simulink model "RobotX_SLAMonly"  (R2014a)
settings: Solver=FixedStepDiscrete  StartTime=0.0  StopTime=inf  FixedStep=.25  RelTol=1e-3
undefined symbols (not defined in the file): Com1, Com2, Com3, Com4, DiscIntNeverNeededParam, standard
libraries: xpcseriallib x11, simulink x3, slrtlib x3, dspmtrx3 x2, speedgoatlib x1, speedgoatlib_IO102 x1
(part 1 of 15)
settings Model: BufferReuse=off  Creator=wildcat  LastModifiedBy=wildcat
settings SolverCC: EnableConcurrentExecution=on
settings DataIOCC: SignalLoggingSaveFormat=ModelDataLogs
settings OptimizationCC: BlockReduction=off  OptimizeBlockIOStorage=off  BufferReuse=off  GlobalBufferReuse=off  ExpressionFolding=off  LocalBlockOutputs=off
settings DebuggingCC: UnderspecifiedInitializationDetection=Classic  StateNameClashWarn=warning
settings HardwareCC: ProdIntDivRoundTo=Zero  ProdEndianess=LittleEndian  ProdHWDeviceType=Generic->32-bit x86 compatible
settings RTWCC: SystemTargetFile=slrt.tlc  TemplateMakefile=slrt_default_tmf  Description=Simulink Real-Time  ProcessScript=slrt_make_rtw_hook  RTWCompilerOptimization=On
settings SimulinkRealTimeCC: GeneratePreprocessorConditionals=Disable all  EnableShiftOperators=on

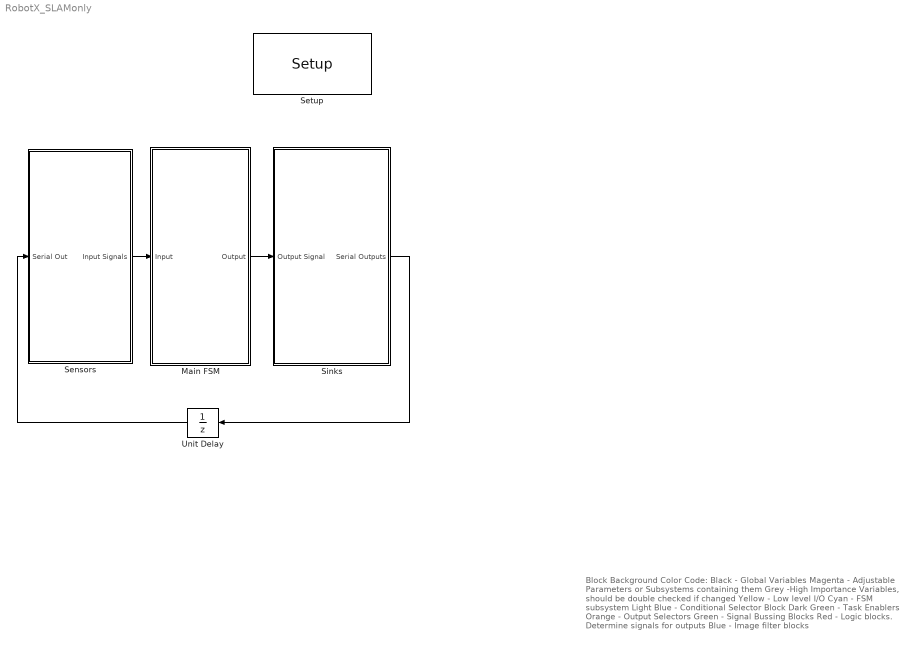
== system RobotX_SLAMonly ==
  note: Block Background Color Code:
      | Black - Global Variables
      | Magenta - Adjustable Parameters or Subsystems containing them
      | Grey -High Importance Variables, should be double checked if changed
      | Yellow - Low level I/O
      | Cyan - FSM subsystem
      | Light Blue - Conditional Selector Block
      | Dark Green - Task Enablers
      | Orange - Output Selectors
      | Green - Signal Bussing Blocks
      | Red - Logic blocks. Determine signals for outputs
      | Blue - Image filter blocks
  Main FSM : Subsystem
  Sensors : Subsystem
  Setup : speedgoatlib_IO102/Setup  group=Digital output setup  id=1  range=+-5V  cal=off  pciSlot=-1  adChannelMode=Multiple-channel (enter number of channels below)  adChannel=16  adCoupling=Differential  daChannel=[1,2,3,4]  daReset=[1]  daInitValue=[0]  diChannel=[1,2,3,4,5,6,7,8]  doChannel=[1,2,3,4,5,6,7,8]  doReset=[1]  doInitValue=[0]
  Sinks : Subsystem
  Unit Delay : UnitDelay  SampleTime=-1
  wires:
  Main FSM/1(Output) -> Sinks/1(Output Signal)
  Sensors/1(Input Signals) -> Main FSM/1(Input)
  Sinks/1(Serial Outputs) -> Unit Delay/1
  Unit Delay/1 -> Sensors/1(Serial Out)

== system RobotX_SLAMonly/Main FSM ==
  Input : Inport
  Angles : dspmtrx3/Submatrix  RowSpan=All rows  RowStartMode=First  RowStartIndex=1  RowEndMode=Last  RowEndIndex=1  ColSpan=One column  ColStartMode=Last  ColStartIndex=1  ColEndMode=Last  ColEndIndex=1
  Bus Selector2 : BusSelector  OutputSignals=Navigation Message.On/Off/RC/Auto
  Distances : dspmtrx3/Submatrix  RowSpan=All rows  RowStartMode=First  RowStartIndex=1  RowEndMode=Last  RowEndIndex=1  ColSpan=One column  ColStartMode=First  ColStartIndex=1  ColEndMode=Last  ColEndIndex=1
  Initialization : Subsystem
  Main Enabler : MATLAB Function  TreatAsAtomicUnit=on
  Multiport Switch : MultiPortSwitch
  Path : Subsystem  TreatAsAtomicUnit=on
  RCHold : Subsystem
  SLAM : Subsystem
  "Scope " : slrtlib/Displays and Logging/Scope   scopeno=1  scopetype=File  autostart=on  viewmode=Graphical redraw  formatstr='%15.6f'  grid=on  ylimits=[0,0]  nosamples=28800  noprepostsamples=0  interleave=1  triggermode=FreeRun  triggersignal=1  trigsignalfromport=off  triggerlevel=0.0  triggerslope=Either  triggerscope=1  triggersample=0  filename=lmD1_<%%%>.dat  mode=Lazy  writesize=512  autorestart=on  dynamicfilemode=on  maxwritefilesize=512*1024^2
  Scope 1 : slrtlib/Displays and Logging/Scope   scopeno=2  scopetype=File  autostart=on  viewmode=Graphical redraw  formatstr='%15.6f'  grid=on  ylimits=[0,0]  nosamples=28800  noprepostsamples=0  interleave=1  triggermode=FreeRun  triggersignal=1  trigsignalfromport=off  triggerlevel=0.0  triggerslope=Either  triggerscope=1  triggersample=0  filename=lmA1_<%%%>.dat  mode=Lazy  writesize=512  autorestart=on  dynamicfilemode=on  maxwritefilesize=512*1024^2
  Unit Delay : UnitDelay  SampleTime=-1
  Output : Outport
  wires:
  Input/1 -> SLAM/1(Sensors), Path/1(Sensors), RCHold/1(Sensors), Initialization/1(Sensors), Bus Selector2/1
  Bus Selector2/1 -> Main Enabler/1(OnOffRCAuto)  "<On/Off/RC/Auto>"
  Initialization/1(Outputs) -> Multiport Switch/2
  Path/1(Outputs) -> Multiport Switch/3
  RCHold/1(Outputs) -> Multiport Switch/4
  Main Enabler/2(initEn) -> Initialization/Enable
  Main Enabler/3(pathEn) -> Path/Enable
  Main Enabler/4(RCEn) -> RCHold/Enable
  Main Enabler/1(taskSelector) -> Multiport Switch/1
  Multiport Switch/1 -> Output/1
  Initialization/2(Finished) -> Unit Delay/1  "Init Fin"
  Unit Delay/1 -> Main Enabler/2(initFin)
  SLAM/1(SLAM Map) -> Angles/1, Distances/1
  Distances/1 -> "Scope "/1
  Angles/1 -> Scope 1/1

== system RobotX_SLAMonly/Sensors ==
  Serial Out : Inport
  Serial In : Subsystem
  Input Signals : Outport
  wires:
  Serial In/1(Serial In) -> Input Signals/1  "Sensors"
  Serial Out/1 -> Serial In/1(Serial Out)

== system RobotX_SLAMonly/Sinks ==
  Output Signal : Inport
  Bus Selector : BusSelector  OutputSignals=Outputs
  data log : Subsystem  Commented=on
  Serial Outputs : Outport
  wires:
  Output Signal/1 -> Bus Selector/1
  Bus Selector/1 -> Serial Outputs/1  "<Outputs>"

== system RobotX_SLAMonly/Main FSM/Initialization ==
  Sensors : Inport
  Enable : EnablePort  ShowOutputPort=on
  Compare To Constant : simulink/Logic and Bit Operations/Compare To Constant  relop=>=  const=50  OutDataTypeStr=boolean
  Data Type Conversion : DataTypeConversion  OutDataTypeStr=double
  Discrete-Time Integrator : DiscreteIntegrator  SampleTime=-1  ICPrevOutput=DiscIntNeverNeededParam  ICPrevScaledInput=DiscIntNeverNeededParam
  Output Heirarchy : Subsystem
  Outputs : Outport
  Finished : Outport  Port=2
  wires:
  Sensors/1 -> Output Heirarchy/1(Sensors)
  Output Heirarchy/1(Outputs) -> Outputs/1
  Compare To Constant/1 -> Data Type Conversion/1
  Enable/1 -> Discrete-Time Integrator/1
  Discrete-Time Integrator/1 -> Compare To Constant/1
  Data Type Conversion/1 -> Finished/1

== system RobotX_SLAMonly/Main FSM/Path ==
  note: Through Gate
  Sensors : Inport
  Enable : EnablePort  ShowOutputPort=on
  A Star (Held Length) : MATLAB Function  TreatAsAtomicUnit=on
  Bus Selector : BusSelector  OutputSignals=Navigation Message.Pose.X,Navigation Message.Pose.Y,Navigation Message.Pose.Psi
  Bus Selector1 : BusSelector  OutputSignals=Navigation Message.Velocity.u
  Calculate Times : MATLAB Function  TreatAsAtomicUnit=on
  Constant : Constant  Value=3
  Constant1 : Constant  Value=[3558, 662; 3625, 652; 3577, 568; 3614, 558]
  Constant2 : Constant  Value=[10, 5; 15, 26; 28, 19; 15, 8; 50, 30]
  Discrete-Time Integrator : DiscreteIntegrator  SampleTime=-1  ICPrevOutput=DiscIntNeverNeededParam  ICPrevScaledInput=DiscIntNeverNeededParam
  Map Grid (Held Length) : MATLAB Function  TreatAsAtomicUnit=on
  Output Reassign : Subsystem
  Path To Trajectory : MATLAB Function  TreatAsAtomicUnit=on
  Outputs : Outport
  wires:
  Output Reassign/1(Outputs) -> Outputs/1
  Enable/1 -> Discrete-Time Integrator/1
  Map Grid (Held Length)/1(relPose) -> A Star (Held Length)/1(relPose), Path To Trajectory/2(relPose)
  Map Grid (Held Length)/2(obGrid) -> A Star (Held Length)/2(obGrid)
  Map Grid (Held Length)/3(targetPt) -> A Star (Held Length)/3(targetPt)
  A Star (Held Length)/1(Path) -> Path To Trajectory/3(Path)
  Map Grid (Held Length)/4(nodes) -> Path To Trajectory/4(nodes)
  Constant/1 -> Map Grid (Held Length)/1(exitGate)
  Constant1/1 -> Map Grid (Held Length)/2(NEDcorners)
  Bus Selector/2 -> Map Grid (Held Length)/4(Y)  "<Y>"
  Bus Selector/3 -> Map Grid (Held Length)/5(Psi)  "<Psi>"
  Constant2/1 -> Map Grid (Held Length)/6(NEDlandmarks)
  Bus Selector/1 -> Map Grid (Held Length)/3(X)  "<X>"
  Path To Trajectory/2(trajectory) -> Calculate Times/1(pts)
  Bus Selector1/1 -> Calculate Times/2(u)  "<u>"
  Path To Trajectory/1(valid) -> Output Reassign/1("Valid ")
  Calculate Times/1(Data) -> Output Reassign/2(Data)
  Sensors/1 -> Output Reassign/3(Sensors), Bus Selector1/1, Bus Selector/1
  Discrete-Time Integrator/1 -> Path To Trajectory/1(time)

== system RobotX_SLAMonly/Main FSM/RCHold ==
  Sensors : Inport
  Enable : EnablePort
  Bus Selector : BusSelector  Commented=on  OutputSignals=LCM Message.Pose.X,LCM Message.Pose.Y,LCM Message.Pose.Psi
  Output Heirarchy : Subsystem  Commented=on
  Output Heirarchy1 : Subsystem
  Set Pose : MATLAB Function  Commented=on  TreatAsAtomicUnit=on
  Outputs : Outport
  wires:
  Output Heirarchy1/1(Outputs) -> Outputs/1
  Bus Selector/1 -> Set Pose/1(X)  "<X>"
  Bus Selector/3 -> Set Pose/3(Psi)  "<Psi>"
  Bus Selector/2 -> Set Pose/2(Y)  "<Y>"
  Set Pose/1(Data) -> Output Heirarchy/1(Data)
  Sensors/1 -> Output Heirarchy1/1(Sensors), Bus Selector/1

== system RobotX_SLAMonly/Main FSM/SLAM ==
  Sensors : Inport
  Any Landmark Change : MATLAB Function  TreatAsAtomicUnit=on
  Any State Change : MATLAB Function  TreatAsAtomicUnit=on
  Bus Selector : BusSelector  OutputSignals=Navigation Message,Lidar Data Input
  Bus Selector1 : BusSelector  OutputSignals=Landmarks.Distances,Landmarks.Angles
  Bus Selector2 : BusSelector  OutputSignals=Pose
  Detect Change : simulink/Logic and Bit Operations/Detect Change  vinit=0  InputProcessing=Inherited  OutDataTypeStr=boolean
  Detect Change1 : simulink/Logic and Bit Operations/Detect Change  vinit=0  InputProcessing=Inherited  OutDataTypeStr=boolean
  Landmark Organizer : MATLAB Function  TreatAsAtomicUnit=on
  Models for prediction : Subsystem
  SLAM enabled : Subsystem  TreatAsAtomicUnit=on
  inputselection : Subsystem
  SLAM Map : Outport
  wires:
  Sensors/1 -> Bus Selector/1
  Bus Selector/1 -> Models for prediction/1(Nav Messages), Bus Selector2/1, Detect Change/1  "<Navigation Message>"
  Bus Selector/2 -> Bus Selector1/1  "<Lidar Data Input>"
  Bus Selector1/1 -> Landmark Organizer/1(Distances)  "<Distances>"
  Bus Selector1/2 -> Landmark Organizer/2(Angles)  "<Angles>"
  Landmark Organizer/1(lm_data) -> SLAM enabled/2(lm_data), Detect Change1/1
  Detect Change/1 -> Any State Change/1(u)
  Detect Change1/1 -> Any Landmark Change/1(u)
  Any Landmark Change/1(y) -> SLAM enabled/Enable, inputselection/3(Landmarkchange)
  Bus Selector2/1 -> inputselection/2(xypsi)  "<Pose>"
  Any State Change/1(y) -> inputselection/1(controlchange)
  SLAM enabled/2(part_positions) -> inputselection/4(part_positions)
  inputselection/1(last particle positions) -> Models for prediction/2(xypsi150)
  Models for prediction/1(xypsioutput) -> inputselection/5(xypsi150), SLAM enabled/1(pre_past_positions)
  SLAM enabled/1(mpa) -> SLAM Map/1  "SLAM Map"

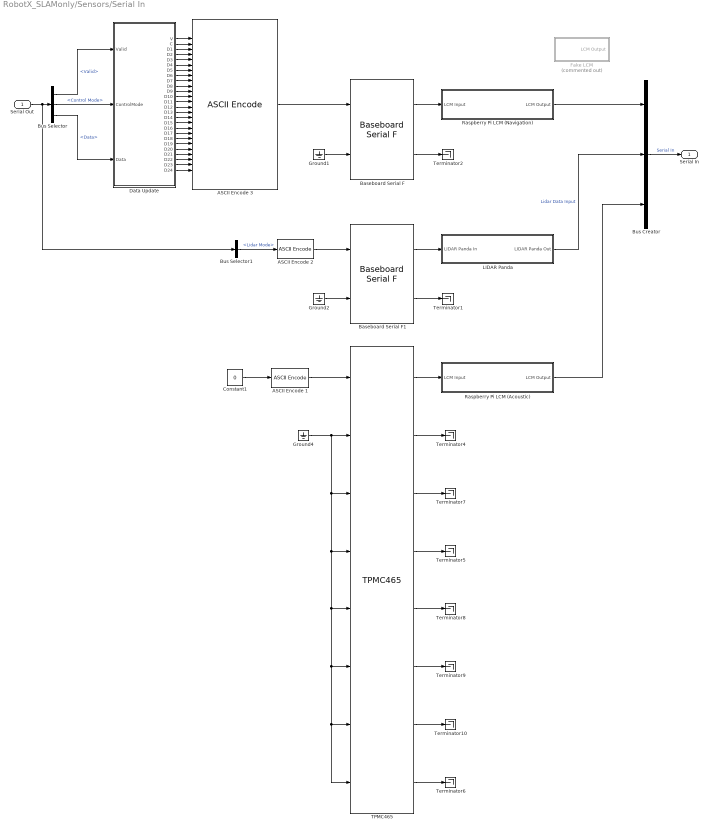
== system RobotX_SLAMonly/Sensors/Serial In ==
  Serial Out : Inport
  " Raspberry Pi LCM (Acoustic)" : Subsystem
  " Raspberry Pi LCM (Navigation)" : Subsystem
  ASCII Encode 1 : xpcseriallib/ASCII Encode   format="{\"Activate\":%d} \\r\\n"  nvars=1  maxlength=20  vartypes={ 'double' }
  ASCII Encode 2 : xpcseriallib/ASCII Encode   format=SGTask:%d \r\n  nvars=1  maxlength=128  vartypes={ 'double' }
  ASCII Encode 3 : xpcseriallib/ASCII Encode   format="{\"Valid\":%d,\"Mode\":%d,\"A\":%f,\"B\":%f,\"C\":%f,\"D\":%f,\"E\":%f,\"F\":%f,\"G\":%f,\"H\":%f,\"I\":%f,\"J\":%f,\"K\":%f,\"L\":%f,\"M\":%f,\"N\":%f,\"O\":%f,\"P\":%f,\"Q\":%f,\"R\":%f,\"S\":%f,\"T\":%f,\"U\":%f,\"V\":%f,\"W\":%f,\"X\":%f} \\r\\n"  nvars=26  maxlength=450  vartypes={ 'double' }
  Baseboard Serial F : xpcseriallib/Mainboard/Baseboard Serial F  group=Basic Setup  port=1  irqnum=4  saddr1=0x3f8  saddr2=0x3e8  config=Com1/Com3  baud1=115200  parity1=Even  ndata1=7  nstop1=1  fifomode1=64 deep  rlevel1=quarter full  automode1=on  xmtfifosize1=1024  xmtdatatype1=8 bit uint null terminated  rcvfifosize1=1024  baud2=115200  parity2=Even  ndata2=7  nstop2=1  fifomode2=64 deep  rlevel2=1  automode2=on  xmtfifosize2=1024  xmtdatatype2=8 bit uint null terminated  rcvfifosize2=1024
  Baseboard Serial F1 : xpcseriallib/Mainboard/Baseboard Serial F  group=Basic Setup  port=2  irqnum=4  saddr1=0x3f8  saddr2=0x3e8  config=Com2/Com4  baud1=115200  parity1=Even  ndata1=7  nstop1=1  fifomode1=64 deep  rlevel1=quarter full  automode1=on  xmtfifosize1=1024  xmtdatatype1=8 bit uint null terminated  rcvfifosize1=1024  baud2=115200  parity2=Even  ndata2=7  nstop2=1  fifomode2=64 deep  rlevel2=quarter full  automode2=on  xmtfifosize2=1024  xmtdatatype2=8 bit uint null terminated  rcvfifosize2=1024
  Bus Creator : BusCreator  Inputs=3
  Bus Selector : BusSelector  OutputSignals=Navigation Outputs.Valid,Navigation Outputs.Control Mode,Navigation Outputs.Data
  Bus Selector1 : BusSelector  OutputSignals=Lidar Mode
  Constant1 : Constant  Value=0  VectorParams1D=off
  Data Update : MATLAB Function  TreatAsAtomicUnit=on
  Fake LCM : Subsystem  Commented=on
  Ground1 : Ground
  Ground2 : Ground
  Ground4 : Ground
  LIDAR Panda : Subsystem
  TPMC465 : speedgoatlib/IO504/TPMC465  group=Basic Setup  port=2  irqnum=9  slot=-1  transceiver1=RS232 (max 921.6kb/s)  standard1=on  baud1=115200  bauddivisor1=1  sampling1=16x (standard)  prescale1=off  parity1=Even  ndata1=7  nstop1=1  rlevel1=half full (32)  hwmode1=none  swmode1=none  xonchar1=17  xoffchar1=19  rs485auto1=off  rs485delay1=0  xmtfifosize1=1024  xmtdatatype1=8 bit uint null terminated  rcvfifosize1=1024  transceiver2=RS232 (max 921.6kb/s)  standard2=on  baud2=115200  bauddivisor2=1  sampling2=16x (standard)  prescale2=off  parity2=None  ndata2=8  nstop2=1  rlevel2=half full (32)  hwmode2=none  swmode2=none  xonchar2=17  xoffchar2=19  rs485auto2=off  rs485delay2=0  xmtfifosize2=1024  xmtdatatype2=8 bit uint null terminated  rcvfifosize2=1024  transceiver3=RS232 (max 921.6kb/s)  standard3=on  baud3=115200  bauddivisor3=1  sampling3=16x (standard)  prescale3=off  parity3=None  ndata3=8  nstop3=1  rlevel3=half full (32)  hwmode3=none  swmode3=none  xonchar3=17  xoffchar3=19  rs485auto3=off  rs485delay3=0  xmtfifosize3=1024  xmtdatatype3=8 bit uint null terminated  rcvfifosize3=1024  transceiver4=RS232 (max 921.6kb/s)  standard4=on  baud4=115200  bauddivisor4=1  sampling4=16x (standard)  prescale4=off  parity4=None  ndata4=8  nstop4=1  rlevel4=half full (32)  hwmode4=none  swmode4=none  xonchar4=17  xoffchar4=19  rs485auto4=off  rs485delay4=0  xmtfifosize4=1024  xmtdatatype4=8 bit uint null terminated  rcvfifosize4=1024  transceiver5=RS232 (max 921.6kb/s)  standard5=on  baud5=115200  bauddivisor5=1  sampling5=16x (standard)  prescale5=off  parity5=None  ndata5=8  nstop5=1  rlevel5=1  hwmode5=none  swmode5=none  xonchar5=17  xoffchar5=19  rs485auto5=off  rs485delay5=0  xmtfifosize5=1024  xmtdatatype5=8 bit uint null terminated  rcvfifosize5=1024  transceiver6=RS232 (max 921.6kb/s)  standard6=on  baud6=115200  bauddivisor6=1  sampling6=16x (standard)  prescale6=off  parity6=None  ndata6=8  nstop6=1  rlevel6=1  hwmode6=none  swmode6=none  xonchar6=17  xoffchar6=19  rs485auto6=off  rs485delay6=0  xmtfifosize6=1024  xmtdatatype6=8 bit uint null terminated  rcvfifosize6=1024  transceiver7=RS232 (max 921.6kb/s)  standard7=on  baud7=115200  bauddivisor7=1  sampling7=16x (standard)  prescale7=off  parity7=None  ndata7=8  nstop7=1  rlevel7=1  hwmode7=none  swmode7=none  xonchar7=17  xoffchar7=19  rs485auto7=off  rs485delay7=0  xmtfifosize7=1024  xmtdatatype7=8 bit uint null terminated  rcvfifosize7=1024  transceiver8=RS232 (max 921.6kb/s)  standard8=on  baud8=115200  bauddivisor8=1  sampling8=16x (standard)  prescale8=off  parity8=None  ndata8=8  nstop8=1  rlevel8=1  hwmode8=none  swmode8=none  xonchar8=17  xoffchar8=19  rs485auto8=off  rs485delay8=0  xmtfifosize8=1024  xmtdatatype8=8 bit uint null terminated  rcvfifosize8=1024
  Terminator{1..2,4..10} (9 alike) : Terminator
  Serial In : Outport
  wires:
  Bus Creator/1 -> Serial In/1  "Serial In"
  Baseboard Serial F1/1 -> LIDAR Panda/1(LIDAR Panda In)
  Serial Out/1 -> Bus Selector1/1, Bus Selector/1
  Baseboard Serial F/1 -> " Raspberry Pi LCM (Navigation)"/1(LCM Input)
  TPMC465/1 -> " Raspberry Pi LCM (Acoustic)"/1(LCM Input)
  ASCII Encode 3/1 -> Baseboard Serial F/1
  " Raspberry Pi LCM (Navigation)"/1(LCM Output) -> Bus Creator/1
  ASCII Encode 1/1 -> TPMC465/1
  Data Update/9(D7) -> ASCII Encode 3/9
  Data Update/11(D9) -> ASCII Encode 3/11
  Data Update/3(D1) -> ASCII Encode 3/3
  Data Update/6(D4) -> ASCII Encode 3/6
  Data Update/7(D5) -> ASCII Encode 3/7
  Data Update/2(C) -> ASCII Encode 3/2
  Data Update/5(D3) -> ASCII Encode 3/5
  Data Update/4(D2) -> ASCII Encode 3/4
  Data Update/13(D11) -> ASCII Encode 3/13
  Data Update/14(D12) -> ASCII Encode 3/14
  Data Update/1(V) -> ASCII Encode 3/1
  Data Update/12(D10) -> ASCII Encode 3/12
  Data Update/10(D8) -> ASCII Encode 3/10
  Data Update/8(D6) -> ASCII Encode 3/8
  Bus Selector/1 -> Data Update/1(Valid)  "<Valid>"
  Bus Selector/2 -> Data Update/2(ControlMode)  "<Control Mode>"
  Bus Selector/3 -> Data Update/3(Data)  "<Data>"
  Data Update/24(D22) -> ASCII Encode 3/24
  Data Update/26(D24) -> ASCII Encode 3/26
  Data Update/18(D16) -> ASCII Encode 3/18
  Data Update/23(D21) -> ASCII Encode 3/23
  Data Update/22(D20) -> ASCII Encode 3/22
  Data Update/21(D19) -> ASCII Encode 3/21
  Data Update/19(D17) -> ASCII Encode 3/19
  Data Update/17(D15) -> ASCII Encode 3/17
  Data Update/16(D14) -> ASCII Encode 3/16
  Data Update/25(D23) -> ASCII Encode 3/25
  Data Update/20(D18) -> ASCII Encode 3/20
  Data Update/15(D13) -> ASCII Encode 3/15
  " Raspberry Pi LCM (Acoustic)"/1(LCM Output) -> Bus Creator/3
  Baseboard Serial F/2 -> Terminator2/1
  Ground1/1 -> Baseboard Serial F/2
  ASCII Encode 2/1 -> Baseboard Serial F1/1
  LIDAR Panda/1(LIDAR Panda Out) -> Bus Creator/2  "Lidar Data Input"
  TPMC465/7 -> Terminator10/1
  TPMC465/5 -> Terminator8/1
  TPMC465/6 -> Terminator9/1
  TPMC465/3 -> Terminator7/1
  TPMC465/2 -> Terminator4/1
  TPMC465/4 -> Terminator5/1
  TPMC465/8 -> Terminator6/1
  Ground4/1 -> TPMC465/2, TPMC465/3, TPMC465/4, TPMC465/5, TPMC465/6, TPMC465/7, TPMC465/8
  Baseboard Serial F1/2 -> Terminator1/1
  Ground2/1 -> Baseboard Serial F1/2
  Bus Selector1/1 -> ASCII Encode 2/1  "<Lidar Mode>"
  Constant1/1 -> ASCII Encode 1/1

== system RobotX_SLAMonly/Sinks/data log ==
  note: need to play with the boat to figure out how this works properly
  Output signal : Inport
  "Scope " : slrtlib/Displays and Logging/Scope   scopeno=1  scopetype=File  autostart=on  viewmode=Graphical redraw  formatstr='%15.6f'  grid=on  ylimits=[0,0]  nosamples=250  noprepostsamples=0  interleave=1  triggermode=Signal triggering  triggersignal=1  trigsignalfromport=on  triggerlevel=1  triggerslope=Rising  triggerscope=1  triggersample=0  filename=data.dat  mode=Lazy  writesize=512  autorestart=off  dynamicfilemode=off  maxwritefilesize=512*1024^2
  wires:
  Output signal/1 -> ?

== system RobotX_SLAMonly/Main FSM/Initialization/Output Heirarchy ==
  Sensors : Inport
  Acoustic Active : Constant  Value=0
  Bus Creator1 : BusCreator  Inputs=3
  Bus Creator2 : BusCreator  Inputs=3
  Bus Creator4 : BusCreator  Inputs=2
  Constant : Constant  Value=0
  Constant1 : Constant  Value=0
  Constant2 : Constant  Value=zeros(24,1)
  Lidar Mode : Constant  Value=0
  Outputs : Outport
  wires:
  Sensors/1 -> Bus Creator4/2  "Sensors"
  Bus Creator4/1 -> Outputs/1  "Output Signals"
  Constant/1 -> Bus Creator1/1  "Valid"
  Constant1/1 -> Bus Creator1/2  "Control Mode"
  Constant2/1 -> Bus Creator1/3  "Data"
  Bus Creator1/1 -> Bus Creator2/1  "Navigation Outputs"
  Acoustic Active/1 -> Bus Creator2/2  "Acoustic Active"
  Lidar Mode/1 -> Bus Creator2/3  "Lidar Mode"
  Bus Creator2/1 -> Bus Creator4/1  "Outputs"

== system RobotX_SLAMonly/Main FSM/Path/Output Reassign ==
  "Valid " : Inport
  Data : Inport  Port=2
  Sensors : Inport  Port=3
  Acoustic Active : Constant
  Bus Creator2 : BusCreator  Inputs=3
  Bus Creator3 : BusCreator  Inputs=3
  Bus Creator5 : BusCreator  Inputs=2
  Constant3 : Constant
  Lidar Mode : Constant
  Outputs : Outport
  wires:
  Sensors/1 -> Bus Creator5/2  "Sensors"
  Bus Creator5/1 -> Outputs/1  "Output Signals"
  "Valid "/1 -> Bus Creator2/1  "Valid"
  Constant3/1 -> Bus Creator2/2  "Control Mode"
  Data/1 -> Bus Creator2/3  "Data"
  Bus Creator2/1 -> Bus Creator3/1  "Navigation Outputs"
  Acoustic Active/1 -> Bus Creator3/2  "Acoustic Active"
  Lidar Mode/1 -> Bus Creator3/3  "Lidar Mode"
  Bus Creator3/1 -> Bus Creator5/1  "Outputs"

== system RobotX_SLAMonly/Main FSM/RCHold/Output Heirarchy ==
  Data : Inport
  Sensors1 : Inport  Port=2
  Acoustic Active : Constant  Value=0
  Bus Creator2 : BusCreator  Inputs=3
  Bus Creator3 : BusCreator  Inputs=3
  Bus Creator5 : BusCreator  Inputs=2
  Constant : Constant
  Constant3 : Constant
  Lidar Mode : Constant
  Outputs : Outport
  wires:
  Sensors1/1 -> Bus Creator5/2  "Sensors"
  Bus Creator5/1 -> Outputs/1  "Output Signals"
  Constant/1 -> Bus Creator2/1  "Valid"
  Constant3/1 -> Bus Creator2/2  "Control Mode"
  Data/1 -> Bus Creator2/3  "Data"
  Bus Creator2/1 -> Bus Creator3/1  "Navigation Outputs"
  Acoustic Active/1 -> Bus Creator3/2  "Acoustic Active"
  Lidar Mode/1 -> Bus Creator3/3  "Lidar Mode"
  Bus Creator3/1 -> Bus Creator5/1  "Outputs"

== system RobotX_SLAMonly/Main FSM/RCHold/Output Heirarchy1 ==
  Sensors : Inport
  Acoustic Active : Constant  Value=0
  Bus Creator1 : BusCreator  Inputs=3
  Bus Creator2 : BusCreator  Inputs=3
  Bus Creator4 : BusCreator  Inputs=2
  Constant : Constant  Value=0
  Constant1 : Constant  Value=2
  Constant2 : Constant  Value=zeros(24,1)
  Lidar Mode : Constant
  Outputs : Outport
  wires:
  Sensors/1 -> Bus Creator4/2  "Sensors"
  Bus Creator4/1 -> Outputs/1  "Output Signals"
  Constant/1 -> Bus Creator1/1  "Valid"
  Constant1/1 -> Bus Creator1/2  "Control Mode"
  Constant2/1 -> Bus Creator1/3  "Data"
  Bus Creator1/1 -> Bus Creator2/1  "Navigation Outputs"
  Acoustic Active/1 -> Bus Creator2/2  "Acoustic Active"
  Lidar Mode/1 -> Bus Creator2/3  "Lidar Mode"
  Bus Creator2/1 -> Bus Creator4/1  "Outputs"

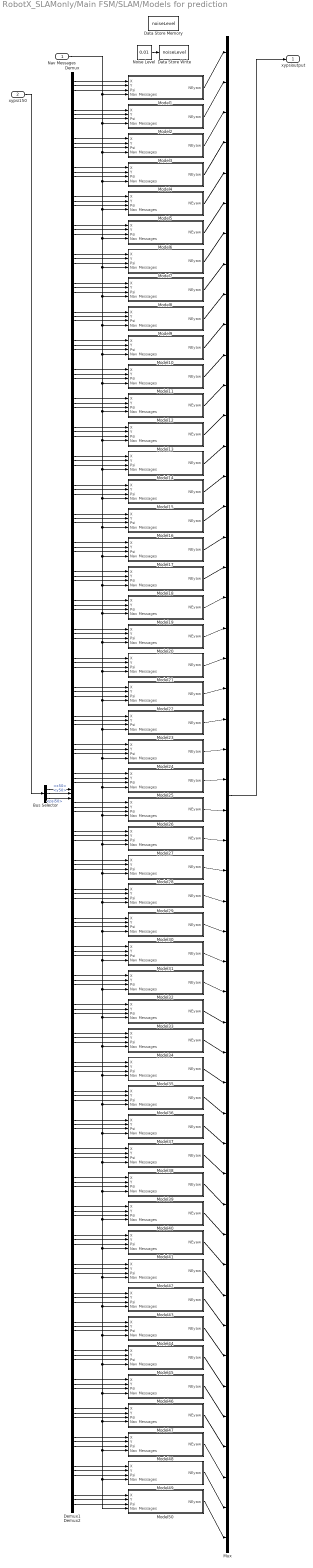
== system RobotX_SLAMonly/Main FSM/SLAM/Models for prediction ==
  Nav Messages : Inport
  xypsi150 : Inport  Port=2
  Bus Selector : BusSelector  OutputSignals=x50,y50,psi50
  Data Store Memory : DataStoreMemory  DataStoreName=noiseLevel  ReadBeforeWriteMsg=warning  WriteAfterWriteMsg=warning  WriteAfterReadMsg=warning
  Data Store Write : DataStoreWrite  DataStoreName=noiseLevel
  Demux : Demux  Outputs=50
  Demux1 : Demux  Outputs=50
  Demux2 : Demux  Outputs=50
  Model1 : Subsystem
  Model10 : Subsystem
  Model11 : Subsystem
  Model12 : Subsystem
  Model13 : Subsystem
  Model14 : Subsystem
  Model15 : Subsystem
  Model16 : Subsystem
  Model17 : Subsystem
  Model18 : Subsystem
  Model19 : Subsystem
  Model2 : Subsystem
  Model20 : Subsystem
  Model21 : Subsystem
  Model22 : Subsystem
  Model23 : Subsystem
  Model24 : Subsystem
  Model25 : Subsystem
  Model26 : Subsystem
  Model27 : Subsystem
  Model28 : Subsystem
  Model29 : Subsystem
  Model3 : Subsystem
  Model30 : Subsystem
  Model31 : Subsystem
  Model32 : Subsystem
  Model33 : Subsystem
  Model34 : Subsystem
  Model35 : Subsystem
  Model36 : Subsystem
  Model37 : Subsystem
  Model38 : Subsystem
  Model39 : Subsystem
  Model4 : Subsystem
  Model40 : Subsystem
  Model41 : Subsystem
  Model42 : Subsystem
  Model43 : Subsystem
  Model44 : Subsystem
  Model45 : Subsystem
  Model46 : Subsystem
  Model47 : Subsystem
  Model48 : Subsystem
  Model49 : Subsystem
  Model5 : Subsystem
  Model50 : Subsystem
  Model6 : Subsystem
  Model7 : Subsystem
  Model8 : Subsystem
  Model9 : Subsystem
  Mux : Mux  Inputs=50
  Noise Level : Constant  Value=0.01
  xypsioutput : Outport  PortDimensions=150
  wires:
  Noise Level/1 -> Data Store Write/1
  Demux/1 -> Model1/1(X)
  Demux1/1 -> Model1/2(Y)
  Demux2/1 -> Model1/3(Psi)
  Demux/2 -> Model2/1(X)
  Demux1/2 -> Model2/2(Y)
  Demux2/2 -> Model2/3(Psi)
  Demux/3 -> Model3/1(X)
  Demux1/3 -> Model3/2(Y)
  Demux2/3 -> Model3/3(Psi)
  Demux/4 -> Model4/1(X)
  Demux1/4 -> Model4/2(Y)
  Demux2/4 -> Model4/3(Psi)
  Demux/5 -> Model5/1(X)
  Demux1/5 -> Model5/2(Y)
  Demux2/5 -> Model5/3(Psi)
  Demux/6 -> Model6/1(X)
  Demux1/6 -> Model6/2(Y)
  Demux2/6 -> Model6/3(Psi)
  Nav Messages/1 -> Model1/4(Nav Messages), Model2/4(Nav Messages), Model3/4(Nav Messages), Model4/4(Nav Messages), Model5/4(Nav Messages), Model6/4(Nav Messages), Model7/4(Nav Messages), Model8/4(Nav Messages), Model9/4(Nav Messages), Model10/4(Nav Messages), Model11/4(Nav Messages), Model12/4(Nav Messages), Model13/4(Nav Messages), Model14/4(Nav Messages), Model15/4(Nav Messages), Model16/4(Nav Messages), Model17/4(Nav Messages), Model18/4(Nav Messages), Model19/4(Nav Messages), Model20/4(Nav Messages), Model21/4(Nav Messages), Model22/4(Nav Messages), Model23/4(Nav Messages), Model24/4(Nav Messages), Model25/4(Nav Messages), Model26/4(Nav Messages), Model27/4(Nav Messages), Model28/4(Nav Messages), Model29/4(Nav Messages), Model30/4(Nav Messages), Model31/4(Nav Messages), Model32/4(Nav Messages), Model33/4(Nav Messages), Model34/4(Nav Messages), Model35/4(Nav Messages), Model36/4(Nav Messages), Model37/4(Nav Messages), Model38/4(Nav Messages), Model39/4(Nav Messages), Model40/4(Nav Messages), Model41/4(Nav Messages), Model42/4(Nav Messages), Model43/4(Nav Messages), Model44/4(Nav Messages), Model45/4(Nav Messages), Model46/4(Nav Messages), Model47/4(Nav Messages), Model48/4(Nav Messages), Model50/4(Nav Messages), Model49/4(Nav Messages)
  Demux2/15 -> Model15/3(Psi)
  Demux1/15 -> Model15/2(Y)
  Demux/15 -> Model15/1(X)
  Demux2/14 -> Model14/3(Psi)
  Demux1/14 -> Model14/2(Y)
  Demux/14 -> Model14/1(X)
  Demux2/13 -> Model13/3(Psi)
  Demux1/13 -> Model13/2(Y)
  Demux/13 -> Model13/1(X)
  Demux2/12 -> Model12/3(Psi)
  Demux1/12 -> Model12/2(Y)
  Demux/12 -> Model12/1(X)
  Demux2/11 -> Model11/3(Psi)
  Demux1/11 -> Model11/2(Y)
  Demux/11 -> Model11/1(X)
  Demux2/10 -> Model10/3(Psi)
  Demux1/10 -> Model10/2(Y)
  Demux/10 -> Model10/1(X)
  Demux2/9 -> Model9/3(Psi)
  Demux1/9 -> Model9/2(Y)
  Demux/9 -> Model9/1(X)
  Demux2/8 -> Model8/3(Psi)
  Demux1/8 -> Model8/2(Y)
  Demux/8 -> Model8/1(X)
  Demux2/7 -> Model7/3(Psi)
  Demux1/7 -> Model7/2(Y)
  Demux/7 -> Model7/1(X)
  Demux/16 -> Model16/1(X)
  Demux1/16 -> Model16/2(Y)
  Demux2/16 -> Model16/3(Psi)
  Demux/17 -> Model17/1(X)
  Demux1/17 -> Model17/2(Y)
  Demux2/17 -> Model17/3(Psi)
  Demux/18 -> Model18/1(X)
  Demux1/18 -> Model18/2(Y)
  Demux2/18 -> Model18/3(Psi)
  Demux/19 -> Model19/1(X)
  Demux1/19 -> Model19/2(Y)
  Demux2/19 -> Model19/3(Psi)
  Demux/20 -> Model20/1(X)
  Demux1/20 -> Model20/2(Y)
  Demux2/20 -> Model20/3(Psi)
  Demux/21 -> Model21/1(X)
  Demux1/21 -> Model21/2(Y)
  Demux2/21 -> Model21/3(Psi)
  Demux/22 -> Model22/1(X)
  Demux1/22 -> Model22/2(Y)
  Demux2/22 -> Model22/3(Psi)
  Demux/23 -> Model23/1(X)
  Demux1/23 -> Model23/2(Y)
  Demux2/23 -> Model23/3(Psi)
  Demux/24 -> Model24/1(X)
  Demux1/24 -> Model24/2(Y)
  Demux2/24 -> Model24/3(Psi)
  Demux/25 -> Model25/1(X)
  Demux1/25 -> Model25/2(Y)
  Demux2/25 -> Model25/3(Psi)
  Demux/26 -> Model26/1(X)
  Demux1/26 -> Model26/2(Y)
  Demux2/26 -> Model26/3(Psi)
  Demux/27 -> Model27/1(X)
  Demux1/27 -> Model27/2(Y)
  Demux2/27 -> Model27/3(Psi)
  Demux/28 -> Model28/1(X)
  Demux1/28 -> Model28/2(Y)
  Demux2/28 -> Model28/3(Psi)
  Demux/29 -> Model29/1(X)
  Demux1/29 -> Model29/2(Y)
  Demux2/29 -> Model29/3(Psi)
  Demux/30 -> Model30/1(X)
  Demux1/30 -> Model30/2(Y)
  Demux2/30 -> Model30/3(Psi)
  Demux/31 -> Model31/1(X)
  Demux1/31 -> Model31/2(Y)
  Demux2/31 -> Model31/3(Psi)
  Demux/32 -> Model32/1(X)
  Demux1/32 -> Model32/2(Y)
  Demux2/32 -> Model32/3(Psi)
  Demux/33 -> Model33/1(X)
  Demux1/33 -> Model33/2(Y)
  Demux2/33 -> Model33/3(Psi)
  Demux/34 -> Model34/1(X)
  Demux1/34 -> Model34/2(Y)
  Demux2/34 -> Model34/3(Psi)
  Demux/35 -> Model35/1(X)
  Demux1/35 -> Model35/2(Y)
  Demux2/35 -> Model35/3(Psi)
  Demux/36 -> Model36/1(X)
  Demux1/36 -> Model36/2(Y)
  Demux2/36 -> Model36/3(Psi)
  Demux/37 -> Model37/1(X)
  Demux1/37 -> Model37/2(Y)
  Demux2/37 -> Model37/3(Psi)
  Demux/38 -> Model38/1(X)
  Demux1/38 -> Model38/2(Y)
  Demux2/38 -> Model38/3(Psi)
  Demux/39 -> Model39/1(X)
  Demux1/39 -> Model39/2(Y)
  Demux2/39 -> Model39/3(Psi)
  Demux/40 -> Model40/1(X)
  Demux1/40 -> Model40/2(Y)
  Demux2/40 -> Model40/3(Psi)
  Demux/41 -> Model41/1(X)
  Demux1/41 -> Model41/2(Y)
  Demux2/41 -> Model41/3(Psi)
  Demux/42 -> Model42/1(X)
  Demux1/42 -> Model42/2(Y)
  Demux2/42 -> Model42/3(Psi)
  Demux/43 -> Model43/1(X)
  Demux1/43 -> Model43/2(Y)
  Demux2/43 -> Model43/3(Psi)
  Demux/44 -> Model44/1(X)
  Demux1/44 -> Model44/2(Y)
  Demux2/44 -> Model44/3(Psi)
  Demux/45 -> Model45/1(X)
  Demux1/45 -> Model45/2(Y)
  Demux2/45 -> Model45/3(Psi)
  Demux/46 -> Model46/1(X)
  Demux1/46 -> Model46/2(Y)
  Demux2/46 -> Model46/3(Psi)
  Demux/47 -> Model47/1(X)
  Demux1/47 -> Model47/2(Y)
  Demux2/47 -> Model47/3(Psi)
  Demux/48 -> Model48/1(X)
  Demux1/48 -> Model48/2(Y)
  Demux2/48 -> Model48/3(Psi)
  Demux/49 -> Model49/1(X)
  Demux1/49 -> Model49/2(Y)
  Demux2/49 -> Model49/3(Psi)
  Demux/50 -> Model50/1(X)
  Demux1/50 -> Model50/2(Y)
  Demux2/50 -> Model50/3(Psi)
  xypsi150/1 -> Bus Selector/1
  Bus Selector/1 -> Demux/1  "<x50>"
  Bus Selector/2 -> Demux1/1  "<y50>"
  Bus Selector/3 -> Demux2/1  "<psi50>"
  Model27/1(NEyaw) -> Mux/27
  Model26/1(NEyaw) -> Mux/26
  Model25/1(NEyaw) -> Mux/25
  Model24/1(NEyaw) -> Mux/24
  Model28/1(NEyaw) -> Mux/28
  Model23/1(NEyaw) -> Mux/23
  Model21/1(NEyaw) -> Mux/21
  Model30/1(NEyaw) -> Mux/30
  Model29/1(NEyaw) -> Mux/29
  Model22/1(NEyaw) -> Mux/22
  Model40/1(NEyaw) -> Mux/40
  Model33/1(NEyaw) -> Mux/33
  Model36/1(NEyaw) -> Mux/36
  Model38/1(NEyaw) -> Mux/38
  Model37/1(NEyaw) -> Mux/37
  Model35/1(NEyaw) -> Mux/35
  Model39/1(NEyaw) -> Mux/39
  Model31/1(NEyaw) -> Mux/31
  Model32/1(NEyaw) -> Mux/32
  Model34/1(NEyaw) -> Mux/34
  Model2/1(NEyaw) -> Mux/2
  Model5/1(NEyaw) -> Mux/5
  Model3/1(NEyaw) -> Mux/3
  Model4/1(NEyaw) -> Mux/4
  Model19/1(NEyaw) -> Mux/19
  Model13/1(NEyaw) -> Mux/13
  Model14/1(NEyaw) -> Mux/14
  Model12/1(NEyaw) -> Mux/12
  Model16/1(NEyaw) -> Mux/16
  Model17/1(NEyaw) -> Mux/17
  Model18/1(NEyaw) -> Mux/18
  Model20/1(NEyaw) -> Mux/20
  Model11/1(NEyaw) -> Mux/11
  Model15/1(NEyaw) -> Mux/15
  Model10/1(NEyaw) -> Mux/10
  Model8/1(NEyaw) -> Mux/8
  Model9/1(NEyaw) -> Mux/9
  Model7/1(NEyaw) -> Mux/7
  Model6/1(NEyaw) -> Mux/6
  Model48/1(NEyaw) -> Mux/48
  Model42/1(NEyaw) -> Mux/42
  Model49/1(NEyaw) -> Mux/49
  Model47/1(NEyaw) -> Mux/47
  Model50/1(NEyaw) -> Mux/50
  Model43/1(NEyaw) -> Mux/43
  Model45/1(NEyaw) -> Mux/45
  Model44/1(NEyaw) -> Mux/44
  Model46/1(NEyaw) -> Mux/46
  Model41/1(NEyaw) -> Mux/41
  Model1/1(NEyaw) -> Mux/1
  Mux/1 -> xypsioutput/1

== system RobotX_SLAMonly/Main FSM/SLAM/SLAM enabled ==
  pre_past_positions : Inport
  lm_data : Inport  Port=2
  Enable : EnablePort
  slammed : MATLAB Function  TreatAsAtomicUnit=on
  mpa : Outport
  part_positions : Outport  Port=2
  wires:
  lm_data/1 -> slammed/1(lm_data)
  pre_past_positions/1 -> slammed/2(pre_part_positions)
  slammed/1(mpa) -> mpa/1
  slammed/2(part_positions) -> part_positions/1

== system RobotX_SLAMonly/Main FSM/SLAM/inputselection ==
  controlchange : Inport
  xypsi : Inport  Port=2
  Landmarkchange : Inport  Port=3
  part_positions : Inport  Port=4
  xypsi150 : Inport  Port=5
  Bus Creator : BusCreator  Inputs=3
  Delay{,1..4} (5 alike) : Delay  DelayLength=1  InitialCondition=0
  MATLAB Function : MATLAB Function  TreatAsAtomicUnit=on
  last particle positions : Outport
  wires:
  Delay/1 -> MATLAB Function/4(part_positions)
  Delay1/1 -> MATLAB Function/3(xypsi)
  Delay2/1 -> MATLAB Function/5(xypsi150)
  Delay4/1 -> MATLAB Function/1(Landmarkchange)
  Delay3/1 -> MATLAB Function/2(controlchange)
  controlchange/1 -> Delay3/1
  xypsi/1 -> Delay1/1
  part_positions/1 -> Delay/1
  Landmarkchange/1 -> Delay4/1
  xypsi150/1 -> Delay2/1
  MATLAB Function/2(y50) -> Bus Creator/2  "y50"
  MATLAB Function/3(psi50) -> Bus Creator/3  "psi50"
  MATLAB Function/1(x50) -> Bus Creator/1  "x50"
  Bus Creator/1 -> last particle positions/1  "last particle positions"

== system RobotX_SLAMonly/Sensors/Serial In/ Raspberry Pi LCM (Acoustic) ==
  LCM Input : Inport
  ASCII Decode 6 : xpcseriallib/ASCII Decode   format=Deploy:%1u, Elapsed:%g, Bearing1:%g Bearing2:%g \r\n  nvars=4  vartypes={}
  Bus Creator : BusCreator  Inputs=2
  Bus Creator1 : BusCreator  Inputs=3
  FIFO ASCII read 1 : xpcseriallib/FIFO ASCII read   header={'Deploy:'}  term=[13 10]  hold=Zero output if no new data  enable=off  maxsize=1024  outputtype=8 bit uint null terminated  sampletime=-1
  LCM Output : Outport
  wires:
  LCM Input/1 -> FIFO ASCII read 1/1
  FIFO ASCII read 1/1 -> ASCII Decode 6/1
  ASCII Decode 6/3 -> Bus Creator/1  "Horizontal Bearing"
  ASCII Decode 6/4 -> Bus Creator/2  "Vertical Bearing"
  Bus Creator/1 -> Bus Creator1/3  "Bearings"
  ASCII Decode 6/2 -> Bus Creator1/2  "Elapsed Time"
  ASCII Decode 6/1 -> Bus Creator1/1  "Deployed"
  Bus Creator1/1 -> LCM Output/1  "Acoustic Message"

== system RobotX_SLAMonly/Sensors/Serial In/ Raspberry Pi LCM (Navigation) ==
  LCM Input : Inport
  ASCII Decode 6 : xpcseriallib/ASCII Decode   format=P1:%f P2:%f P3:%f V1:%f V2:%f V3:%f E1:%f E2:%f E3:%f Pt1:%f Pt2:%f St1:%f St2:%f Start:%f Elapsed:%f RC:%d \r\n  nvars=16  vartypes={}
  Bus Creator1 : BusCreator  Inputs=3
  Bus Creator2 : BusCreator  Inputs=3
  Bus Creator3 : BusCreator  Inputs=3
  Bus Creator4 : BusCreator  Inputs=8
  Bus Creator5 : BusCreator  Inputs=2
  Bus Creator6 : BusCreator  Inputs=2
  Data Type Conversion : DataTypeConversion  OutDataTypeStr=double
  FIFO ASCII read 1 : xpcseriallib/FIFO ASCII read   header={'P1:'}  term=[13 10]  hold=Zero output if no new data  enable=off  maxsize=1024  outputtype=8 bit uint null terminated  sampletime=-1
  LCM Output : Outport
  wires:
  LCM Input/1 -> FIFO ASCII read 1/1
  FIFO ASCII read 1/1 -> ASCII Decode 6/1
  Bus Creator4/1 -> LCM Output/1  "Navigation Message"
  ASCII Decode 6/1 -> Bus Creator1/1  "X"
  ASCII Decode 6/2 -> Bus Creator1/2  "Y"
  ASCII Decode 6/3 -> Bus Creator1/3  "Psi"
  Bus Creator1/1 -> Bus Creator4/1  "Pose"
  ASCII Decode 6/4 -> Bus Creator2/1  "u"
  ASCII Decode 6/5 -> Bus Creator2/2  "v"
  Bus Creator2/1 -> Bus Creator4/2  "Velocity"
  ASCII Decode 6/7 -> Bus Creator3/1  "Roll"
  ASCII Decode 6/8 -> Bus Creator3/2  "Pitch"
  ASCII Decode 6/9 -> Bus Creator3/3  "Yaw"
  Bus Creator3/1 -> Bus Creator4/3  "Euler"
  Bus Creator5/1 -> Bus Creator4/4  "Port"
  Bus Creator6/1 -> Bus Creator4/5  "Stbd"
  ASCII Decode 6/12 -> Bus Creator6/1  "StThrust"
  ASCII Decode 6/13 -> Bus Creator6/2  "StAzimuth"
  ASCII Decode 6/10 -> Bus Creator5/1  "PtThrust"
  ASCII Decode 6/11 -> Bus Creator5/2  "PtAzimuth"
  ASCII Decode 6/14 -> Bus Creator4/6  "Start"
  ASCII Decode 6/15 -> Bus Creator4/7  "Elapsed"
  ASCII Decode 6/16 -> Data Type Conversion/1  "On/Off/RC/Auto"
  Data Type Conversion/1 -> Bus Creator4/8  "On/Off/RC/Auto"
  ASCII Decode 6/6 -> Bus Creator2/3  "r"

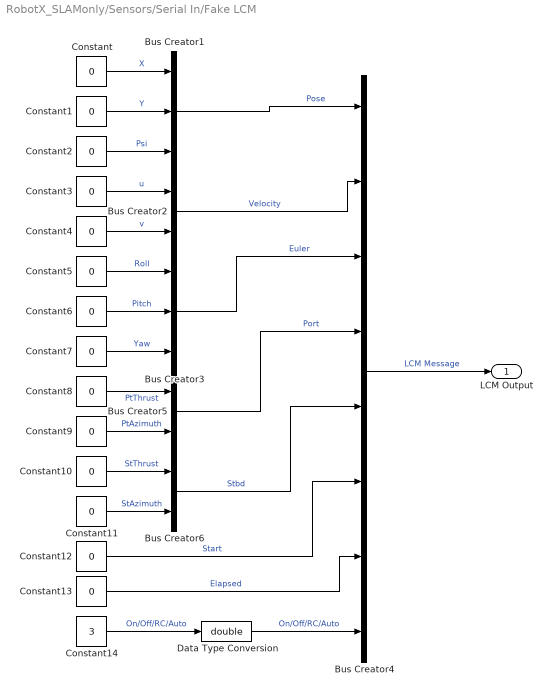
== system RobotX_SLAMonly/Sensors/Serial In/Fake LCM ==
  Bus Creator1 : BusCreator  Inputs=3
  Bus Creator2 : BusCreator  Inputs=2
  Bus Creator3 : BusCreator  Inputs=3
  Bus Creator4 : BusCreator  Inputs=8
  Bus Creator5 : BusCreator  Inputs=2
  Bus Creator6 : BusCreator  Inputs=2
  Constant{,1..13} (14 alike) : Constant  Value=0
  Constant14 : Constant  Value=3
  Data Type Conversion : DataTypeConversion  OutDataTypeStr=double
  LCM Output : Outport
  wires:
  Bus Creator4/1 -> LCM Output/1  "LCM Message"
  Constant/1 -> Bus Creator1/1  "X"
  Constant1/1 -> Bus Creator1/2  "Y"
  Constant2/1 -> Bus Creator1/3  "Psi"
  Bus Creator1/1 -> Bus Creator4/1  "Pose"
  Constant3/1 -> Bus Creator2/1  "u"
  Constant4/1 -> Bus Creator2/2  "v"
  Bus Creator2/1 -> Bus Creator4/2  "Velocity"
  Constant5/1 -> Bus Creator3/1  "Roll"
  Constant6/1 -> Bus Creator3/2  "Pitch"
  Constant7/1 -> Bus Creator3/3  "Yaw"
  Bus Creator3/1 -> Bus Creator4/3  "Euler"
  Bus Creator5/1 -> Bus Creator4/4  "Port"
  Bus Creator6/1 -> Bus Creator4/5  "Stbd"
  Constant10/1 -> Bus Creator6/1  "StThrust"
  Constant11/1 -> Bus Creator6/2  "StAzimuth"
  Constant8/1 -> Bus Creator5/1  "PtThrust"
  Constant9/1 -> Bus Creator5/2  "PtAzimuth"
  Constant12/1 -> Bus Creator4/6  "Start"
  Constant13/1 -> Bus Creator4/7  "Elapsed"
  Constant14/1 -> Data Type Conversion/1  "On/Off/RC/Auto"
  Data Type Conversion/1 -> Bus Creator4/8  "On/Off/RC/Auto"

== system RobotX_SLAMonly/Sensors/Serial In/LIDAR Panda ==
  LIDAR Panda In : Inport
  ASCII Decode 2 : xpcseriallib/ASCII Decode   format=A:%d B:%d C:%d E:%d F:%d G:%d H:%d I:%d J:%d K:%d L:%d M:%d N:%d O:%d P:%d Q:%d R:%d S:%d T:%d U:%d V:%d W:%d X:%d C1:%d C2:%d C3:%d C4:%d P1:%f P2:%f P3:%f P4:%f I1:%d I2:%d I3:%d I4:%d \r\n  nvars=36  vartypes={}
  Bus Creator1 : BusCreator  Inputs=2
  Bus Creator2 : BusCreator  Inputs=3
  Bus Creator3 : BusCreator  Inputs=2
  Data Type Conversion{,1..3} (4 alike) : DataTypeConversion  OutDataTypeStr=double
  "FIFO ASCII read " : xpcseriallib/FIFO ASCII read   header={'A:'}  term=[13 10]  hold=Zero output if no new data  enable=off  maxsize=1024  outputtype=8 bit uint null terminated  sampletime=-1
  Mux : Mux  Inputs=12
  Mux1 : Mux
  Mux2 : Mux  Inputs=12
  Mux3 : Mux
  Mux4 : Mux
  LIDAR Panda Out : Outport
  wires:
  LIDAR Panda In/1 -> "FIFO ASCII read "/1
  "FIFO ASCII read "/1 -> ASCII Decode 2/1
  ASCII Decode 2/3 -> Mux/3  "Distance"
  ASCII Decode 2/2 -> Mux/2  "Color ID"
  ASCII Decode 2/4 -> Mux/4  "Angle"
  ASCII Decode 2/1 -> Mux/1  "Probability"
  ASCII Decode 2/7 -> Mux/7
  ASCII Decode 2/10 -> Mux/10
  ASCII Decode 2/11 -> Mux/11
  ASCII Decode 2/6 -> Mux/6
  ASCII Decode 2/8 -> Mux/8
  ASCII Decode 2/9 -> Mux/9
  ASCII Decode 2/12 -> Mux/12
  ASCII Decode 2/5 -> Mux/5
  ASCII Decode 2/13 -> Mux2/1
  ASCII Decode 2/15 -> Mux2/3
  ASCII Decode 2/22 -> Mux2/10
  ASCII Decode 2/23 -> Mux2/11
  ASCII Decode 2/17 -> Mux2/5
  ASCII Decode 2/18 -> Mux2/6
  ASCII Decode 2/14 -> Mux2/2
  ASCII Decode 2/24 -> Mux2/12
  ASCII Decode 2/20 -> Mux2/8
  ASCII Decode 2/19 -> Mux2/7
  ASCII Decode 2/21 -> Mux2/9
  ASCII Decode 2/16 -> Mux2/4
  ASCII Decode 2/25 -> Mux1/1
  ASCII Decode 2/28 -> Mux1/4
  ASCII Decode 2/26 -> Mux1/2
  ASCII Decode 2/27 -> Mux1/3
  ASCII Decode 2/30 -> Mux3/2
  ASCII Decode 2/31 -> Mux3/3
  ASCII Decode 2/32 -> Mux3/4
  ASCII Decode 2/29 -> Mux3/1
  ASCII Decode 2/36 -> Mux4/4
  ASCII Decode 2/34 -> Mux4/2
  ASCII Decode 2/35 -> Mux4/3
  ASCII Decode 2/33 -> Mux4/1
  Mux/1 -> Data Type Conversion/1  "Distances"
  Mux2/1 -> Data Type Conversion1/1  "Angles"
  Mux1/1 -> Data Type Conversion2/1  "Color"
  Mux3/1 -> Bus Creator2/2  "Probability"
  Mux4/1 -> Data Type Conversion3/1  "idx"
  Bus Creator1/1 -> Bus Creator3/1  "Landmarks"
  Bus Creator2/1 -> Bus Creator3/2  "Color data"
  Bus Creator3/1 -> LIDAR Panda Out/1
  Data Type Conversion/1 -> Bus Creator1/1  "Distances"
  Data Type Conversion1/1 -> Bus Creator1/2  "Angles"
  Data Type Conversion2/1 -> Bus Creator2/1  "Color"
  Data Type Conversion3/1 -> Bus Creator2/3  "Color"

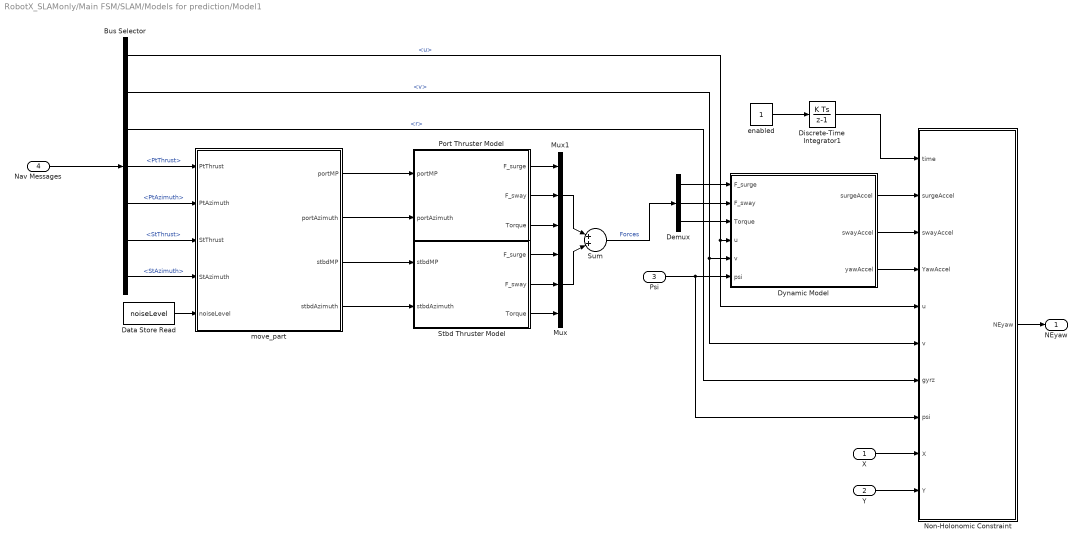
== system RobotX_SLAMonly/Main FSM/SLAM/Models for prediction/Model1 ==
  X : Inport
  Y : Inport  Port=2
  Psi : Inport  Port=3
  Nav Messages : Inport  Port=4
  Bus Selector : BusSelector  OutputSignals=Velocity.u,Velocity.v,Velocity.r,Port.PtThrust,Port.PtAzimuth,Stbd.StThrust,Stbd.StAzimuth
  Data Store Read : DataStoreRead  DataStoreName=noiseLevel
  Demux : Demux  Outputs=3
  Discrete-Time Integrator1 : DiscreteIntegrator  SampleTime=-1  ICPrevOutput=DiscIntNeverNeededParam  ICPrevScaledInput=DiscIntNeverNeededParam
  Dynamic Model : MATLAB Function  TreatAsAtomicUnit=on
  Mux : Mux  Inputs=3
  Mux1 : Mux  Inputs=3
  Non-Holonomic Constraint : MATLAB Function  TreatAsAtomicUnit=on
  Port Thruster Model : MATLAB Function  TreatAsAtomicUnit=on
  Stbd Thruster Model : MATLAB Function  TreatAsAtomicUnit=on
  Sum : Sum  Inputs=|++|
  enabled : Constant
  move_part : MATLAB Function  TreatAsAtomicUnit=on
  NEyaw : Outport
  wires:
  Sum/1 -> Demux/1  "Forces"
  Bus Selector/2 -> Non-Holonomic Constraint/6(v), Dynamic Model/5(v)  "<v>"
  Bus Selector/1 -> Non-Holonomic Constraint/5(u), Dynamic Model/4(u)  "<u>"
  Psi/1 -> Non-Holonomic Constraint/8(psi), Dynamic Model/6(psi)
  Demux/2 -> Dynamic Model/2(F_sway)
  Demux/3 -> Dynamic Model/3(Torque)
  Demux/1 -> Dynamic Model/1(F_surge)
  Mux/1 -> Sum/2
  Stbd Thruster Model/1(F_surge) -> Mux/1
  Stbd Thruster Model/3(Torque) -> Mux/3
  Stbd Thruster Model/2(F_sway) -> Mux/2
  Mux1/1 -> Sum/1
  Port Thruster Model/2(F_sway) -> Mux1/2
  Port Thruster Model/1(F_surge) -> Mux1/1
  Port Thruster Model/3(Torque) -> Mux1/3
  Dynamic Model/1(surgeAccel) -> Non-Holonomic Constraint/2(surgeAccel)
  Dynamic Model/2(swayAccel) -> Non-Holonomic Constraint/3(swayAccel)
  Dynamic Model/3(yawAccel) -> Non-Holonomic Constraint/4(YawAccel)
  Y/1 -> Non-Holonomic Constraint/10(Y)
  X/1 -> Non-Holonomic Constraint/9(X)
  Bus Selector/3 -> Non-Holonomic Constraint/7(gyrz)  "<r>"
  Non-Holonomic Constraint/1(NEyaw) -> NEyaw/1
  enabled/1 -> Discrete-Time Integrator1/1
  Discrete-Time Integrator1/1 -> Non-Holonomic Constraint/1(time)
  Nav Messages/1 -> Bus Selector/1
  Bus Selector/4 -> move_part/1(PtThrust)  "<PtThrust>"
  Bus Selector/5 -> move_part/2(PtAzimuth)  "<PtAzimuth>"
  Bus Selector/7 -> move_part/4(StAzimuth)  "<StAzimuth>"
  Bus Selector/6 -> move_part/3(StThrust)  "<StThrust>"
  move_part/1(portMP) -> Port Thruster Model/1(portMP)
  move_part/2(portAzimuth) -> Port Thruster Model/2(portAzimuth)
  move_part/3(stbdMP) -> Stbd Thruster Model/1(stbdMP)
  move_part/4(stbdAzimuth) -> Stbd Thruster Model/2(stbdAzimuth)
  Data Store Read/1 -> move_part/5(noiseLevel)

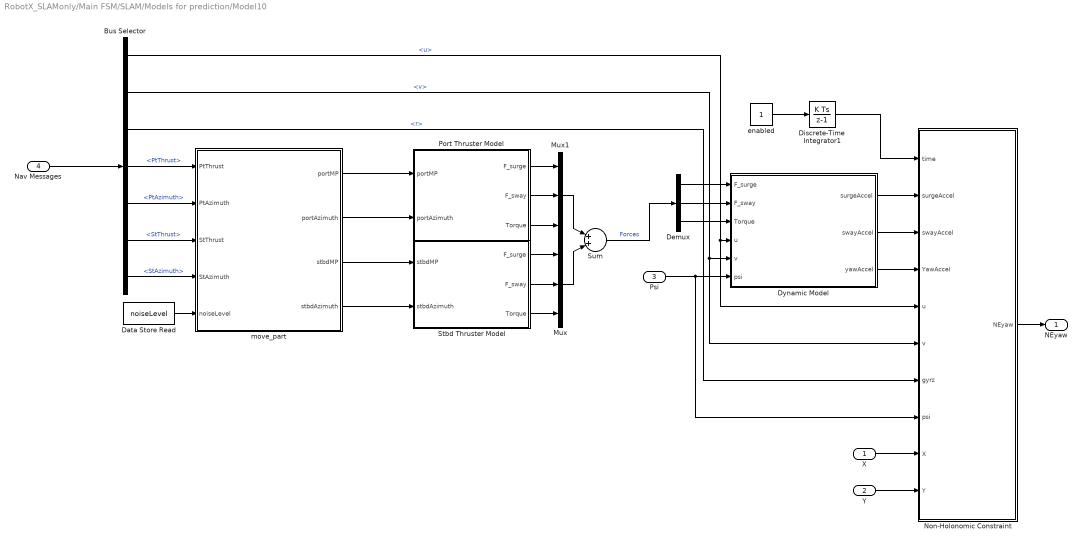
== system RobotX_SLAMonly/Main FSM/SLAM/Models for prediction/Model10 ==
  X : Inport
  Y : Inport  Port=2
  Psi : Inport  Port=3
  Nav Messages : Inport  Port=4
  Bus Selector : BusSelector  OutputSignals=Velocity.u,Velocity.v,Velocity.r,Port.PtThrust,Port.PtAzimuth,Stbd.StThrust,Stbd.StAzimuth
  Data Store Read : DataStoreRead  DataStoreName=noiseLevel
  Demux : Demux  Outputs=3
  Discrete-Time Integrator1 : DiscreteIntegrator  SampleTime=-1  ICPrevOutput=DiscIntNeverNeededParam  ICPrevScaledInput=DiscIntNeverNeededParam
  Dynamic Model : MATLAB Function  TreatAsAtomicUnit=on
  Mux : Mux  Inputs=3
  Mux1 : Mux  Inputs=3
  Non-Holonomic Constraint : MATLAB Function  TreatAsAtomicUnit=on
  Port Thruster Model : MATLAB Function  TreatAsAtomicUnit=on
  Stbd Thruster Model : MATLAB Function  TreatAsAtomicUnit=on
  Sum : Sum  Inputs=|++|
  enabled : Constant
  move_part : MATLAB Function  TreatAsAtomicUnit=on
  NEyaw : Outport
  wires:
  Sum/1 -> Demux/1  "Forces"
  Bus Selector/2 -> Non-Holonomic Constraint/6(v), Dynamic Model/5(v)  "<v>"
  Bus Selector/1 -> Non-Holonomic Constraint/5(u), Dynamic Model/4(u)  "<u>"
  Psi/1 -> Non-Holonomic Constraint/8(psi), Dynamic Model/6(psi)
  Demux/2 -> Dynamic Model/2(F_sway)
  Demux/3 -> Dynamic Model/3(Torque)
  Demux/1 -> Dynamic Model/1(F_surge)
  Mux/1 -> Sum/2
  Stbd Thruster Model/1(F_surge) -> Mux/1
  Stbd Thruster Model/3(Torque) -> Mux/3
  Stbd Thruster Model/2(F_sway) -> Mux/2
  Mux1/1 -> Sum/1
  Port Thruster Model/2(F_sway) -> Mux1/2
  Port Thruster Model/1(F_surge) -> Mux1/1
  Port Thruster Model/3(Torque) -> Mux1/3
  Dynamic Model/1(surgeAccel) -> Non-Holonomic Constraint/2(surgeAccel)
  Dynamic Model/2(swayAccel) -> Non-Holonomic Constraint/3(swayAccel)
  Dynamic Model/3(yawAccel) -> Non-Holonomic Constraint/4(YawAccel)
  Y/1 -> Non-Holonomic Constraint/10(Y)
  X/1 -> Non-Holonomic Constraint/9(X)
  Bus Selector/3 -> Non-Holonomic Constraint/7(gyrz)  "<r>"
  Non-Holonomic Constraint/1(NEyaw) -> NEyaw/1
  enabled/1 -> Discrete-Time Integrator1/1
  Discrete-Time Integrator1/1 -> Non-Holonomic Constraint/1(time)
  Nav Messages/1 -> Bus Selector/1
  Bus Selector/4 -> move_part/1(PtThrust)  "<PtThrust>"
  Bus Selector/5 -> move_part/2(PtAzimuth)  "<PtAzimuth>"
  Bus Selector/7 -> move_part/4(StAzimuth)  "<StAzimuth>"
  Bus Selector/6 -> move_part/3(StThrust)  "<StThrust>"
  move_part/1(portMP) -> Port Thruster Model/1(portMP)
  move_part/2(portAzimuth) -> Port Thruster Model/2(portAzimuth)
  move_part/3(stbdMP) -> Stbd Thruster Model/1(stbdMP)
  move_part/4(stbdAzimuth) -> Stbd Thruster Model/2(stbdAzimuth)
  Data Store Read/1 -> move_part/5(noiseLevel)

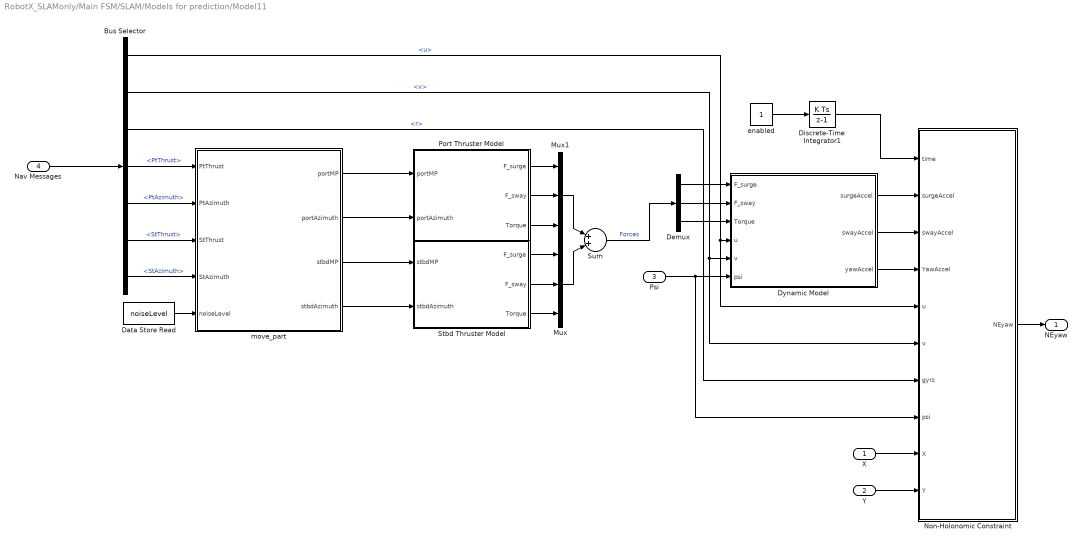
== system RobotX_SLAMonly/Main FSM/SLAM/Models for prediction/Model11 ==
  X : Inport
  Y : Inport  Port=2
  Psi : Inport  Port=3
  Nav Messages : Inport  Port=4
  Bus Selector : BusSelector  OutputSignals=Velocity.u,Velocity.v,Velocity.r,Port.PtThrust,Port.PtAzimuth,Stbd.StThrust,Stbd.StAzimuth
  Data Store Read : DataStoreRead  DataStoreName=noiseLevel
  Demux : Demux  Outputs=3
  Discrete-Time Integrator1 : DiscreteIntegrator  SampleTime=-1  ICPrevOutput=DiscIntNeverNeededParam  ICPrevScaledInput=DiscIntNeverNeededParam
  Dynamic Model : MATLAB Function  TreatAsAtomicUnit=on
  Mux : Mux  Inputs=3
  Mux1 : Mux  Inputs=3
  Non-Holonomic Constraint : MATLAB Function  TreatAsAtomicUnit=on
  Port Thruster Model : MATLAB Function  TreatAsAtomicUnit=on
  Stbd Thruster Model : MATLAB Function  TreatAsAtomicUnit=on
  Sum : Sum  Inputs=|++|
  enabled : Constant
  move_part : MATLAB Function  TreatAsAtomicUnit=on
  NEyaw : Outport
  wires:
  Sum/1 -> Demux/1  "Forces"
  Bus Selector/2 -> Non-Holonomic Constraint/6(v), Dynamic Model/5(v)  "<v>"
  Bus Selector/1 -> Non-Holonomic Constraint/5(u), Dynamic Model/4(u)  "<u>"
  Psi/1 -> Non-Holonomic Constraint/8(psi), Dynamic Model/6(psi)
  Demux/2 -> Dynamic Model/2(F_sway)
  Demux/3 -> Dynamic Model/3(Torque)
  Demux/1 -> Dynamic Model/1(F_surge)
  Mux/1 -> Sum/2
  Stbd Thruster Model/1(F_surge) -> Mux/1
  Stbd Thruster Model/3(Torque) -> Mux/3
  Stbd Thruster Model/2(F_sway) -> Mux/2
  Mux1/1 -> Sum/1
  Port Thruster Model/2(F_sway) -> Mux1/2
  Port Thruster Model/1(F_surge) -> Mux1/1
  Port Thruster Model/3(Torque) -> Mux1/3
  Dynamic Model/1(surgeAccel) -> Non-Holonomic Constraint/2(surgeAccel)
  Dynamic Model/2(swayAccel) -> Non-Holonomic Constraint/3(swayAccel)
  Dynamic Model/3(yawAccel) -> Non-Holonomic Constraint/4(YawAccel)
  Y/1 -> Non-Holonomic Constraint/10(Y)
  X/1 -> Non-Holonomic Constraint/9(X)
  Bus Selector/3 -> Non-Holonomic Constraint/7(gyrz)  "<r>"
  Non-Holonomic Constraint/1(NEyaw) -> NEyaw/1
  enabled/1 -> Discrete-Time Integrator1/1
  Discrete-Time Integrator1/1 -> Non-Holonomic Constraint/1(time)
  Nav Messages/1 -> Bus Selector/1
  Bus Selector/4 -> move_part/1(PtThrust)  "<PtThrust>"
  Bus Selector/5 -> move_part/2(PtAzimuth)  "<PtAzimuth>"
  Bus Selector/7 -> move_part/4(StAzimuth)  "<StAzimuth>"
  Bus Selector/6 -> move_part/3(StThrust)  "<StThrust>"
  move_part/1(portMP) -> Port Thruster Model/1(portMP)
  move_part/2(portAzimuth) -> Port Thruster Model/2(portAzimuth)
  move_part/3(stbdMP) -> Stbd Thruster Model/1(stbdMP)
  move_part/4(stbdAzimuth) -> Stbd Thruster Model/2(stbdAzimuth)
  Data Store Read/1 -> move_part/5(noiseLevel)

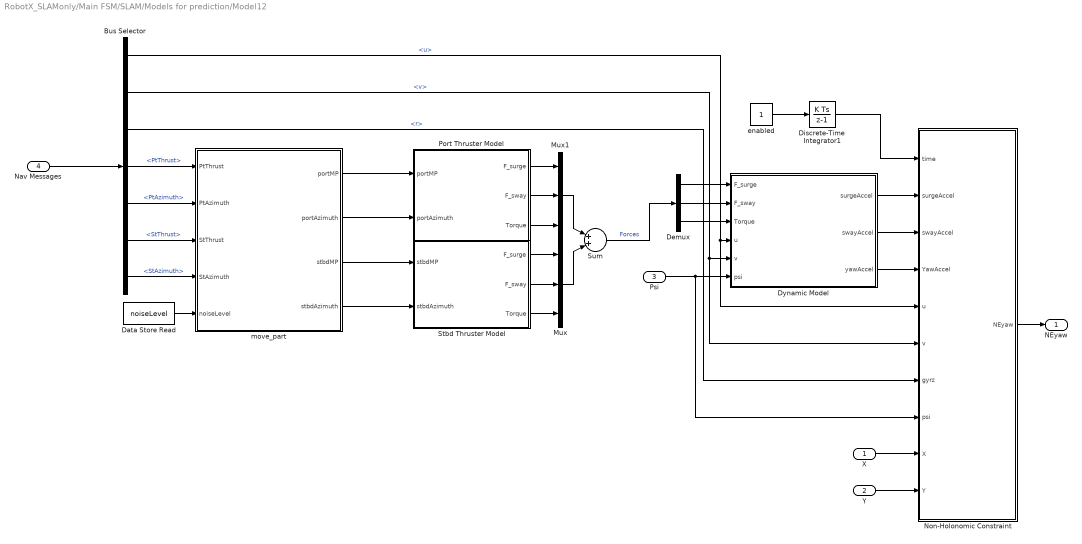
== system RobotX_SLAMonly/Main FSM/SLAM/Models for prediction/Model12 ==
  X : Inport
  Y : Inport  Port=2
  Psi : Inport  Port=3
  Nav Messages : Inport  Port=4
  Bus Selector : BusSelector  OutputSignals=Velocity.u,Velocity.v,Velocity.r,Port.PtThrust,Port.PtAzimuth,Stbd.StThrust,Stbd.StAzimuth
  Data Store Read : DataStoreRead  DataStoreName=noiseLevel
  Demux : Demux  Outputs=3
  Discrete-Time Integrator1 : DiscreteIntegrator  SampleTime=-1  ICPrevOutput=DiscIntNeverNeededParam  ICPrevScaledInput=DiscIntNeverNeededParam
  Dynamic Model : MATLAB Function  TreatAsAtomicUnit=on
  Mux : Mux  Inputs=3
  Mux1 : Mux  Inputs=3
  Non-Holonomic Constraint : MATLAB Function  TreatAsAtomicUnit=on
  Port Thruster Model : MATLAB Function  TreatAsAtomicUnit=on
  Stbd Thruster Model : MATLAB Function  TreatAsAtomicUnit=on
  Sum : Sum  Inputs=|++|
  enabled : Constant
  move_part : MATLAB Function  TreatAsAtomicUnit=on
  NEyaw : Outport
  wires:
  Sum/1 -> Demux/1  "Forces"
  Bus Selector/2 -> Non-Holonomic Constraint/6(v), Dynamic Model/5(v)  "<v>"
  Bus Selector/1 -> Non-Holonomic Constraint/5(u), Dynamic Model/4(u)  "<u>"
  Psi/1 -> Non-Holonomic Constraint/8(psi), Dynamic Model/6(psi)
  Demux/2 -> Dynamic Model/2(F_sway)
  Demux/3 -> Dynamic Model/3(Torque)
  Demux/1 -> Dynamic Model/1(F_surge)
  Mux/1 -> Sum/2
  Stbd Thruster Model/1(F_surge) -> Mux/1
  Stbd Thruster Model/3(Torque) -> Mux/3
  Stbd Thruster Model/2(F_sway) -> Mux/2
  Mux1/1 -> Sum/1
  Port Thruster Model/2(F_sway) -> Mux1/2
  Port Thruster Model/1(F_surge) -> Mux1/1
  Port Thruster Model/3(Torque) -> Mux1/3
  Dynamic Model/1(surgeAccel) -> Non-Holonomic Constraint/2(surgeAccel)
  Dynamic Model/2(swayAccel) -> Non-Holonomic Constraint/3(swayAccel)
  Dynamic Model/3(yawAccel) -> Non-Holonomic Constraint/4(YawAccel)
  Y/1 -> Non-Holonomic Constraint/10(Y)
  X/1 -> Non-Holonomic Constraint/9(X)
  Bus Selector/3 -> Non-Holonomic Constraint/7(gyrz)  "<r>"
  Non-Holonomic Constraint/1(NEyaw) -> NEyaw/1
  enabled/1 -> Discrete-Time Integrator1/1
  Discrete-Time Integrator1/1 -> Non-Holonomic Constraint/1(time)
  Nav Messages/1 -> Bus Selector/1
  Bus Selector/4 -> move_part/1(PtThrust)  "<PtThrust>"
  Bus Selector/5 -> move_part/2(PtAzimuth)  "<PtAzimuth>"
  Bus Selector/7 -> move_part/4(StAzimuth)  "<StAzimuth>"
  Bus Selector/6 -> move_part/3(StThrust)  "<StThrust>"
  move_part/1(portMP) -> Port Thruster Model/1(portMP)
  move_part/2(portAzimuth) -> Port Thruster Model/2(portAzimuth)
  move_part/3(stbdMP) -> Stbd Thruster Model/1(stbdMP)
  move_part/4(stbdAzimuth) -> Stbd Thruster Model/2(stbdAzimuth)
  Data Store Read/1 -> move_part/5(noiseLevel)
